simulink model "Lead_Acid_Battery3"  (R2024b)
settings: Solver=VariableStepAuto  StartTime=0.0  StopTime=36000  RelTol=1e-3
settings Model: Creator=10537  LastModifiedBy=10537

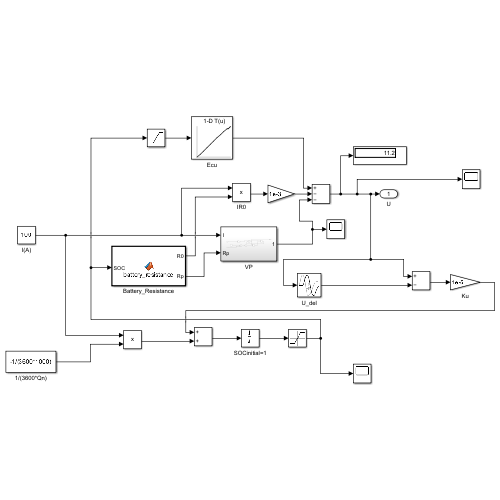
[thumbnail: Simulink's stored preview of the top-level diagram]
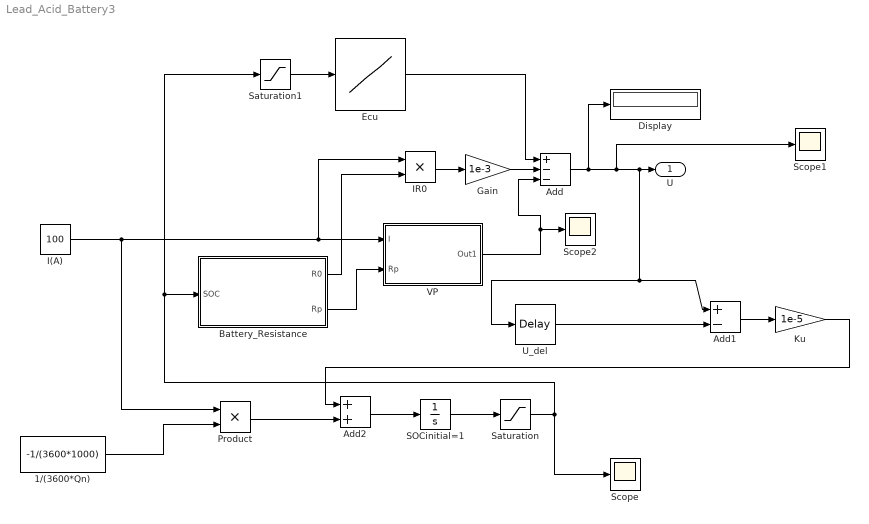
== system Lead_Acid_Battery3 ==
  1/(3600*Qn) : Constant  Value=-1/(3600*1000)
  Add : Sum  Inputs=+--
  Add1 : Sum  Inputs=+-
  Add2 : Sum
  Battery_Resistance : MATLAB Function  TreatAsAtomicUnit=on
  Display : Display
  Ecu : Lookup_n-D  NumberOfTableDimensions=1  BreakpointsForDimension1=[0;0.10000000000000001;0.20000000000000001;0.29999999999999999;0.40000000000000002;0.5;0.59999999999999998;0.69999999999999996;0.80000000000000004;0.90000000000000002;0.92000000000000004;0.93999999999999995;0.95999999999999996;0.97999999999999998;0.98999999999999999;1]  Table=[11.5;11.61;11.76;11.91;12.06;12.2;12.34;12.47;12.6;12.72;12.73;12.74;12.75;12.78;12.8;12.83]  TableDataTypeStr=Inherit: Inherit from 'Table data'  InternalRulePriority=Speed  OutDataTypeStr=Inherit: Inherit via back propagation  RndMeth=Simplest
  Gain : Gain  Gain=1e-3
  I(A) : Constant  Value=100
  IR0 : Product
  Ku : Gain  Gain=1e-5
  Product : Product
  SOCinitial=1 : Integrator  InitialCondition=1
  Saturation : Saturate  UpperLimit=1  LowerLimit=0
  Saturation1 : Saturate  UpperLimit=1  LowerLimit=0
  Scope : Scope
  Scope1 : Scope
  Scope2 : Scope
  U_del : TransportDelay  DelayTime=0.005
  VP : Subsystem
  U : Outport
  wires:
  I(A)/1 -> VP/1(I), IR0/1, Product/1
  Saturation/1 -> Scope/1, Saturation1/1, Battery_Resistance/1(SOC)
  U_del/1 -> Add1/2
  Add1/1 -> Ku/1
  1/(3600*Qn)/1 -> Product/2
  Add2/1 -> SOCinitial=1/1
  Ku/1 -> Add2/1
  Product/1 -> Add2/2
  SOCinitial=1/1 -> Saturation/1
  IR0/1 -> Gain/1
  Gain/1 -> Add/2
  Saturation1/1 -> Ecu/1
  Ecu/1 -> Add/1
  VP/1(Out1) -> Scope2/1, Add/3
  Battery_Resistance/2(Rp) -> VP/2(Rp)
  Battery_Resistance/1(R0) -> IR0/2
  Add/1 -> Scope1/1, U/1, U_del/1, Add1/1, Display/1

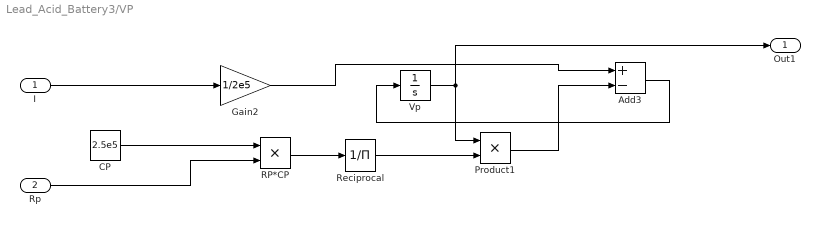
== system Lead_Acid_Battery3/VP ==
  I : Inport
  Rp : Inport  Port=2
  Add3 : Sum  Inputs=+-
  CP : Constant  Value=2.5e5
  Gain2 : Gain  Gain=1/2e5
  Product1 : Product
  RP*CP : Product
  Reciprocal : Product  Inputs=/
  Vp : Integrator
  Out1 : Outport
  wires:
  CP/1 -> RP*CP/1
  I/1 -> Gain2/1
  RP*CP/1 -> Reciprocal/1
  Reciprocal/1 -> Product1/2
  Gain2/1 -> Add3/1
  Add3/1 -> Vp/1
  Vp/1 -> Out1/1, Product1/1
  Product1/1 -> Add3/2
  Rp/1 -> RP*CP/2

== matlab function Lead_Acid_Battery3/Battery_Resistance ==
  data: SOC input; R0 output; Rp output
function [R0, Rp] = battery_resistance(SOC)
    % 电池的欧姆内阻 R0（根据二次曲线拟合）
    a0 = 0.5; a1 = 0.1; a2 = -0.02;  
    R0 = a0 + a1 * SOC + a2 * SOC^2;

    % 电池的极化内阻 Rp（根据指数曲线拟合）
   %c0 = 2.0e-3;
   % c1 = -1.0e-3;
   %c2 =  0.8e-3;
   
   %c3 = -0.3e-3;             % 示例系数（单位：Ω）
   %Rp = c0 + c1*SOC + c2*SOC^2 + c3*SOC^3;
   c3 = -0.3e-3;
   c2 =  0.8e-3;
   c1 = -1.0e-3;
   c0 =  2.0e-3;
   Rp = ((c3*SOC + c2)*SOC + c1)*SOC + c0;
end
